simulink model "ex4_sim3"  (R2017b)
settings: Solver=ode45  StartTime=0.0  StopTime=30  MaxStep=0.001  RelTol=1e-3  EnableMultiTasking=on
undefined symbols (not defined in the file): Ad, As, b, denCth, denCx, dth0, dx0, g, Ie, l, m, Me, numCth, numCx, td, th0, ts, x0
Description:
  | Riccardo Antonello (riccardo.antonello@unipd.it) and Angelo Cenedese (angelo.cenedese@unipd.it)
  | 
  | May 2, 2017
  | 
  | Dept. of Information Engineering, University of Padova
settings Model: Creator=Riccardo  LastModifiedBy=riccardo
settings DataIOCC: LimitDataPoints=on  SaveFormat=Array
settings OptimizationCC: LifeSpan=inf
settings DebuggingCC: AlgebraicLoopMsg=none  SolverPrmCheckMsg=warning  SFUnexpectedBacktrackingDiag=warning  SFNoUnconditionalDefaultTransitionDiag=warning  SFExecutionAtInitializationDiag=none
settings HardwareCC: ProdBitPerPointer=32  ProdBitPerSizeT=32  ProdBitPerPtrDiffT=32  ProdLargestAtomicFloat=None  ProdIntDivRoundTo=Undefined  ProdEndianess=Unspecified  ProdWordSize=32  ProdHWDeviceType=32-bit Generic
settings ModelReferenceCC: PropagateSignalLabelsOutOfModel=off
settings CodeAppCC: StateflowObjectComments=on
settings GRTTargetCC: TargetLangStandard=C89/C90 (ANSI)  GeneratePreprocessorConditionals=Disable all
settings ConfigComp: CovMetricSettings=dw  CovHtmlReporting=on  CovSaveCumulativeToWorkspaceVar=on  CovSaveSingleToWorkspaceVar=on  CovExternalEMLEnable=off  CovSFcnEnable=off

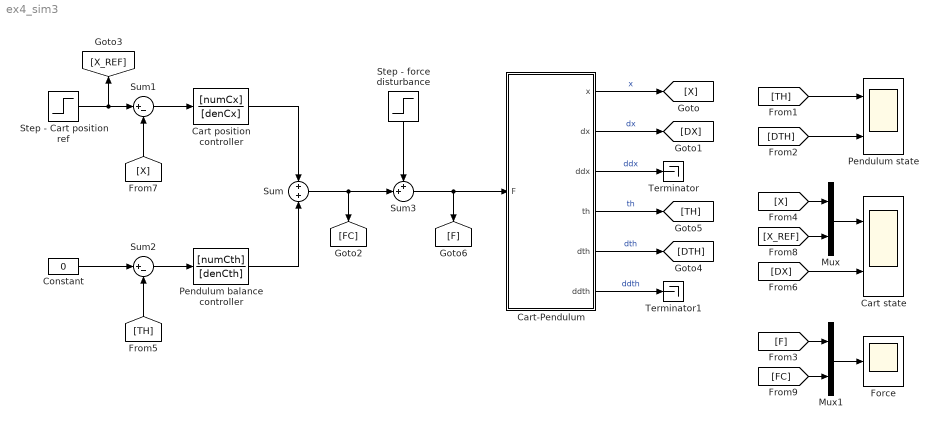
== system ex4_sim3 ==
  Cart position controller : TransferFcn  Numerator=[numCx]  Denominator=[denCx]
  Cart state : Scope  NumInputPorts=2
  Cart-Pendulum : Subsystem
  Constant : Constant  Value=0
  Force : Scope
  Mux : Mux  Inputs=2
  Mux1 : Mux  Inputs=2
  Pendulum balance controller : TransferFcn  Numerator=[numCth]  Denominator=[denCth]
  Pendulum state : Scope  NumInputPorts=2
  Step - Cart position ref : Step  Time=ts  After=As  SampleTime=0
  Step - force disturbance : Step  Time=td  After=Ad  SampleTime=0
  Sum : Sum
  Sum1 : Sum  Inputs=|+-
  Sum2 : Sum  Inputs=|+-
  Sum3 : Sum  Inputs=++|
  Terminator : Terminator
  Terminator1 : Terminator
  wires:
  Cart-Pendulum/1(x) -> [X]  "x"
  Cart-Pendulum/6(ddth) -> Terminator1/1  "ddth"
  Cart-Pendulum/5(dth) -> [DTH]  "dth"
  Cart-Pendulum/4(th) -> [TH]  "th"
  Cart-Pendulum/3(ddx) -> Terminator/1  "ddx"
  Cart-Pendulum/2(dx) -> [DX]  "dx"
  Sum2/1 -> Pendulum balance controller/1
  [TH] -> Sum2/2
  Constant/1 -> Sum2/1
  [TH] -> Pendulum state/1
  [DTH] -> Pendulum state/2
  Sum/1 -> Sum3/2, [FC]
  Pendulum balance controller/1 -> Sum/2
  Cart position controller/1 -> Sum/1
  Sum1/1 -> Cart position controller/1
  Step - Cart position ref/1 -> Sum1/1, [X_REF]
  [X] -> Sum1/2
  [X] -> Mux/1
  Mux/1 -> Cart state/1
  [X_REF] -> Mux/2
  [DX] -> Cart state/2
  Sum3/1 -> Cart-Pendulum/1(F), [F]
  Step - force disturbance/1 -> Sum3/1
  [F] -> Mux1/1
  [FC] -> Mux1/2
  Mux1/1 -> Force/1

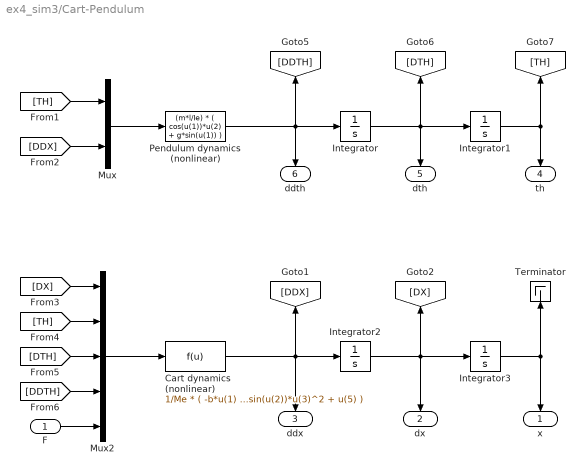
== system ex4_sim3/Cart-Pendulum ==
  F : Inport
  Cart dynamics (nonlinear) : Fcn  Expr=1/Me * ( -b*u(1) + m*l*cos(u(2))*u(4) - m*l*sin(u(2))*u(3)^2 + u(5) )
  Integrator : Integrator  InitialCondition=dth0
  Integrator1 : Integrator  InitialCondition=th0
  Integrator2 : Integrator  InitialCondition=dx0
  Integrator3 : Integrator  InitialCondition=x0
  Mux : Mux  Inputs=2
  Mux2 : Mux  Inputs=5
  Pendulum dynamics (nonlinear) : Fcn  Expr=(m*l/Ie) * ( cos(u(1))*u(2) + g*sin(u(1)) )
  Terminator : Terminator
  x : Outport
  dx : Outport  Port=2
  ddx : Outport  Port=3
  th : Outport  Port=4
  dth : Outport  Port=5
  ddth : Outport  Port=6
  wires:
  Integrator2/1 -> [DX], dx/1, Integrator3/1
  Cart dynamics (nonlinear)/1 -> [DDX], ddx/1, Integrator2/1
  Pendulum dynamics (nonlinear)/1 -> ddth/1, [DDTH], Integrator/1
  Integrator/1 -> dth/1, [DTH], Integrator1/1
  Integrator3/1 -> Terminator/1, x/1
  Integrator1/1 -> [TH], th/1
  Mux/1 -> Pendulum dynamics (nonlinear)/1
  [TH] -> Mux/1
  [DX] -> Mux2/1
  [TH] -> Mux2/2
  [DTH] -> Mux2/3
  [DDTH] -> Mux2/4
  F/1 -> Mux2/5
  Mux2/1 -> Cart dynamics (nonlinear)/1
  [DDX] -> Mux/2
